simulink model "Rainy_Lake_Simulation_Model"  (R2014b)
settings: Solver=ode45  StartTime=0.0  StopTime=40*365  MaxStep=1  RelTol=1e-3
libraries: simulink x1
settings Model: Creator=jeff  LastModifiedBy=jeff
settings SolverCC: ZeroCrossAlgorithm=Adaptive
settings DebuggingCC: IgnoredZcDiagnostic=none

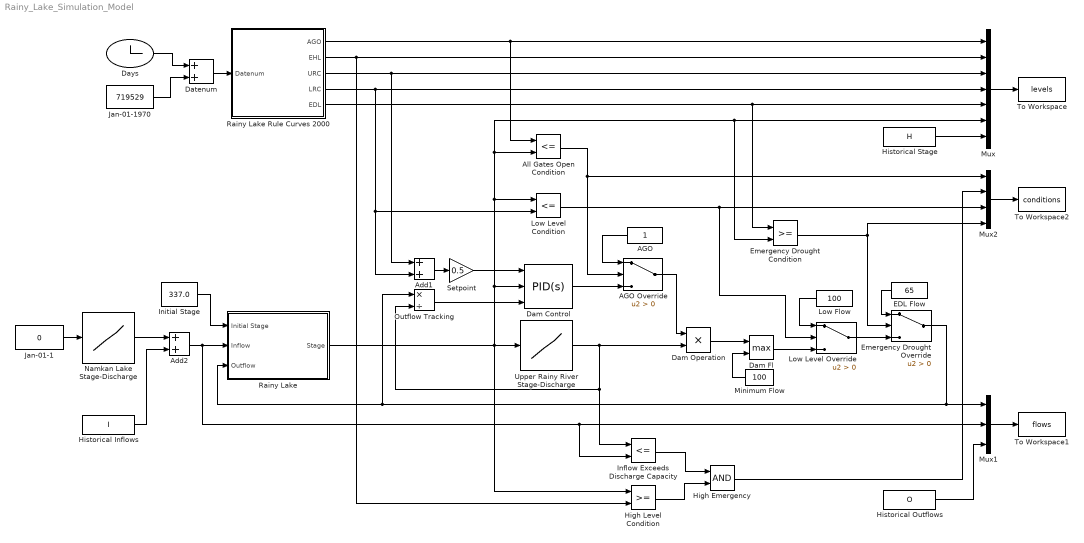
== system Rainy_Lake_Simulation_Model ==
  AGO : Constant
  AGO Override : Switch  Criteria=u2 > Threshold
  Add1 : Sum
  Add2 : Sum
  All Gates Open Condition : RelationalOperator  Operator=<=  OutDataTypeStr=boolean
  Dam Operation : Product
  Dam Control : simulink/Continuous/PID Controller (2DOF)  Controller=PID  TimeDomain=Continuous-time  SampleTime=-1  IntegratorMethod=Forward Euler  FilterMethod=Forward Euler  Form=Parallel  P=-7.76631370345045  I=-0.0682382435942277  D=3.65832815289677  N=2.12291335792304  b=1  c=0  InitialConditionSource=internal  InitialConditionForIntegrator=0  InitialConditionForFilter=0  ExternalReset=none  LimitOutput=on  UpperSaturationLimit=1  LowerSaturationLimit=0  LinearizeAsGain=off  AntiWindupMode=clamping  Kb=1  TrackingMode=on  Kt=1  PParamMin=[]  PParamMax=[]  IParamMin=[]  IParamMax=[]  DParamMin=[]  DParamMax=[]  NParamMin=[]  NParamMax=[]  bParamMin=[]  bParamMax=[]  cParamMin=[]  cParamMax=[]  KbParamMin=[]  KbParamMax=[]  KtParamMin=[]  KtParamMax=[]  POutMin=[]  POutMax=[]  IOutMin=[]  IOutMax=[]  DOutMin=[]  DOutMax=[]  NOutMin=[]  NOutMax=[]  bOutMin=[]  bOutMax=[]  cOutMin=[]  cOutMax=[]  KbOutMin=[]  KbOutMax=[]  KtOutMin=[]  KtOutMax=[]  IntegratorOutMin=[]  IntegratorOutMax=[]  FilterOutMin=[]  FilterOutMax=[]  SumOutMin=[]  SumOutMax=[]  Sum1OutMin=[]  Sum1OutMax=[]  Sum2OutMin=[]  Sum2OutMax=[]  Sum3OutMin=[]  Sum3OutMax=[]  SumI1OutMin=[]  SumI1OutMax=[]  SumI2OutMin=[]  SumI2OutMax=[]  SumI3OutMin=[]  SumI3OutMax=[]  SumDOutMin=[]  SumDOutMax=[]  SaturationOutMin=[]  SaturationOutMax=[]  IntegratorContinuousStateAttributes=''  IntegratorStateMustResolveToSignalObject=off  IntegratorRTWStateStorageClass=Auto  FilterContinuousStateAttributes=''  FilterStateMustResolveToSignalObject=off  FilterRTWStateStorageClass=Auto  DifferentiatorICPrevScaledInput=0  DifferentiatorOutMin=[]  DifferentiatorOutMax=[]  UseFilter=on
  Dam Fl : MinMax  Function=max  Inputs=2
  Datenum : Sum
  Days : Clock
  EDL Flow : Constant  Value=65
  Emergency Drought Condition : RelationalOperator  OutDataTypeStr=boolean
  Emergency Drought Override : Switch  Criteria=u2 > Threshold
  High Emergency : Logic  AllPortsSameDT=off  OutDataTypeStr=boolean
  High Level Condition : RelationalOperator  OutDataTypeStr=boolean
  Historical Inflows : FromWorkspace  VariableName=I  SampleTime=1
  Historical Outflows : FromWorkspace  VariableName=O  SampleTime=1
  Historical Stage : FromWorkspace  VariableName=H  SampleTime=1
  Inflow Exceeds Discharge Capacity : RelationalOperator  Operator=<=  OutDataTypeStr=boolean
  Initial Stage : Constant  Value=337.0
  Jan-01-1 : Constant  Value=0
  Jan-01-1970 : Constant  Value=719529
  Low Flow : Constant  Value=100
  Low Level Condition : RelationalOperator  Operator=<=  OutDataTypeStr=boolean
  Low Level Override : Switch  Criteria=u2 > Threshold
  Minimum Flow : Constant  Value=100
  Mux : Mux  Inputs=7
  Mux1 : Mux  Inputs=3
  Mux2 : Mux
  Namkan Lake Stage-Discharge : Lookup_n-D  NumberOfTableDimensions=1  BreakpointsForDimension1=[335.21, 337.0, 338.0, 338.5, 339.0, 339.5, 340.0, 340.5, 341.0, 341.5, 342.0, 342.5, 343.0]  Table=[0 51 120 173 233 299 373 455 549 659 772 886 999]  ExtrapMethod=Clip  InternalRulePriority=Speed  RndMeth=Simplest  InputSameDT=on
  Outflow Tracking : Product  Inputs=*/
  Rainy Lake : Subsystem
  Rainy Lake Rule Curves 2000 : Subsystem
  Setpoint : Gain  Gain=0.5
  To Workspace : ToWorkspace  VariableName=levels  SaveFormat=Timeseries  SampleTime=-1
  To Workspace1 : ToWorkspace  VariableName=flows  SaveFormat=Timeseries  SampleTime=-1
  To Workspace2 : ToWorkspace  VariableName=conditions  SaveFormat=Timeseries  SampleTime=-1
  Upper Rainy River Stage-Discharge : Lookup_n-D  NumberOfTableDimensions=1  BreakpointsForDimension1="[335.40, 336.00, 336.50, 336.75, 337.00, 337.25,  337.50, 337.75, 338.00, 338.50, 339.00, 339.50, 340.00]"  Table=[0 399 425 443 589 704 792 909 1014 1156 1324 1550 1778]  ExtrapMethod=Clip  InternalRulePriority=Speed  RndMeth=Simplest  InputSameDT=on
  wires:
  Days/1 -> Datenum/1
  Jan-01-1970/1 -> Datenum/2
  Datenum/1 -> Rainy Lake Rule Curves 2000/1(Datenum)
  Mux/1 -> To Workspace/1
  Add1/1 -> Setpoint/1
  Setpoint/1 -> Dam Control/1
  Rainy Lake Rule Curves 2000/3(URC) -> Add1/1, Mux/3
  Rainy Lake Rule Curves 2000/4(LRC) -> Add1/2, Low Level Condition/2, Mux/4
  Upper Rainy River Stage-Discharge/1 -> Outflow Tracking/2, Inflow Exceeds Discharge Capacity/1, Dam Operation/2
  Rainy Lake/1(Stage) -> Emergency Drought Condition/2, Mux/6, All Gates Open Condition/2, Low Level Condition/1, Dam Control/2, High Level Condition/1, Upper Rainy River Stage-Discharge/1
  Initial Stage/1 -> Rainy Lake/1(Initial Stage)
  Mux1/1 -> To Workspace1/1
  Rainy Lake Rule Curves 2000/1(AGO) -> All Gates Open Condition/1, Mux/1
  Historical Stage/1 -> Mux/7
  Historical Outflows/1 -> Mux1/3
  Rainy Lake Rule Curves 2000/2(EHL) -> High Level Condition/2, Mux/2
  Inflow Exceeds Discharge Capacity/1 -> High Emergency/1
  High Level Condition/1 -> High Emergency/2
  Outflow Tracking/1 -> Dam Control/3
  High Emergency/1 -> Mux2/2
  Low Level Condition/1 -> Low Level Override/2, Mux2/3
  Low Flow/1 -> Low Level Override/1
  AGO Override/1 -> Dam Operation/1
  Dam Control/1 -> AGO Override/3
  AGO/1 -> AGO Override/1
  All Gates Open Condition/1 -> AGO Override/2, Mux2/1
  Rainy Lake Rule Curves 2000/5(EDL) -> Emergency Drought Condition/1, Mux/5
  Emergency Drought Override/1 -> Mux1/1, Rainy Lake/3(Outflow), Outflow Tracking/1
  Emergency Drought Condition/1 -> Mux2/4, Emergency Drought Override/2
  EDL Flow/1 -> Emergency Drought Override/1
  Mux2/1 -> To Workspace2/1
  Add2/1 -> Inflow Exceeds Discharge Capacity/2, Mux1/2, Rainy Lake/2(Inflow)
  Namkan Lake Stage-Discharge/1 -> Add2/1
  Historical Inflows/1 -> Add2/2
  Jan-01-1/1 -> Namkan Lake Stage-Discharge/1
  Minimum Flow/1 -> Dam Fl/2
  Dam Operation/1 -> Dam Fl/1
  Dam Fl/1 -> Low Level Override/3
  Low Level Override/1 -> Emergency Drought Override/3

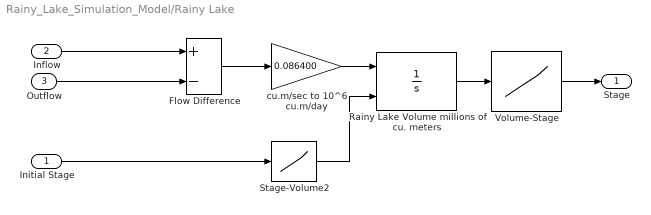
== system Rainy_Lake_Simulation_Model/Rainy Lake ==
  Initial Stage : Inport
  Inflow : Inport  Port=2
  Outflow : Inport  Port=3
  Flow Difference : Sum  Inputs=+-
  Rainy Lake Volume millions of cu. meters : Integrator  InitialConditionSource=external  InitialCondition=1000  LimitOutput=on  LowerSaturationLimit=0  ContinuousStateAttributes='RainyLakeVolume'
  Stage-Volume2 : Lookup_n-D  NumberOfTableDimensions=1  BreakpointsForDimension1=[335.0 336.0 336.5 337.0 337.5 338.0 339.0 340.0]  Table=[112.67 798.00 1176.42 1577.25 2002.06 2450.57 3416.85 4458.97]  InternalRulePriority=Speed  RndMeth=Simplest  InputSameDT=on
  Volume-Stage : Lookup_n-D  NumberOfTableDimensions=1  BreakpointsForDimension1=[112.67 798.00 1176.42 1577.25 2002.06 2450.57 3416.85 4458.97]  Table=[335.0 336.0 336.5 337.0 337.5 338.0 339.0 340.0]  InternalRulePriority=Speed  RndMeth=Simplest  InputSameDT=on
  cu.m/sec to 10^6 cu.m/day : Gain  Gain=0.086400
  Stage : Outport
  wires:
  Outflow/1 -> Flow Difference/2
  Inflow/1 -> Flow Difference/1
  Rainy Lake Volume millions of cu. meters/1 -> Volume-Stage/1
  Stage-Volume2/1 -> Rainy Lake Volume millions of cu. meters/2
  cu.m/sec to 10^6 cu.m/day/1 -> Rainy Lake Volume millions of cu. meters/1
  Initial Stage/1 -> Stage-Volume2/1
  Volume-Stage/1 -> Stage/1
  Flow Difference/1 -> cu.m/sec to 10^6 cu.m/day/1

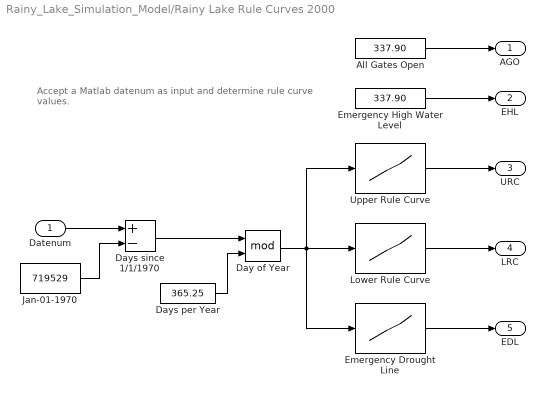
== system Rainy_Lake_Simulation_Model/Rainy Lake Rule Curves 2000 ==
  note: Accept a Matlab datenum as input and determine rule curve values.
  Datenum : Inport
  All Gates Open : Constant  Value=337.90
  Day of Year : Math  Operator=mod  SaturateOnIntegerOverflow=on
  Days per Year : Constant  Value=365.25
  Days since 1/1/1970 : Sum  Inputs=+-
  Emergency Drought Line : Lookup_n-D  NumberOfTableDimensions=1  BreakpointsForDimension1=[0 91 181 182 297 366]  Table=[336.90 336.70 336.70 337.20 337.20 336.90]  InternalRulePriority=Speed  RndMeth=Simplest  InputSameDT=on
  Emergency High Water Level : Constant  Value=337.90
  Jan-01-1970 : Constant  Value=719529
  Lower Rule Curve : Lookup_n-D  NumberOfTableDimensions=1  BreakpointsForDimension1=[0 91 121 152 182 227 335 366]  Table=[337.20 336.70 336.80 337.30 337.50 337.50 337.30 337.20]  InternalRulePriority=Speed  RndMeth=Simplest  InputSameDT=on
  Upper Rule Curve : Lookup_n-D  NumberOfTableDimensions=1  BreakpointsForDimension1=[0 91 121 152 182 227 335 366]  Table="[337.45 337.0  337.40 337.60 337.75 337.75 337.60 337.45]"  InternalRulePriority=Speed  RndMeth=Simplest  InputSameDT=on
  AGO : Outport
  EHL : Outport  Port=2
  URC : Outport  Port=3
  LRC : Outport  Port=4
  EDL : Outport  Port=5
  wires:
  Jan-01-1970/1 -> Days since 1/1/1970/2
  Days since 1/1/1970/1 -> Day of Year/1
  Days per Year/1 -> Day of Year/2
  Day of Year/1 -> Upper Rule Curve/1, Emergency Drought Line/1, Lower Rule Curve/1
  Upper Rule Curve/1 -> URC/1
  Lower Rule Curve/1 -> LRC/1
  Datenum/1 -> Days since 1/1/1970/1
  All Gates Open/1 -> AGO/1
  Emergency Drought Line/1 -> EDL/1
  Emergency High Water Level/1 -> EHL/1
